simulink model "simulink"  (R2022b)
settings: Solver=VariableStepAuto  StartTime=0.0  StopTime=20  RelTol=1e-3
settings Model: Creator=25035  LastModifiedBy=ROG
settings ModelReferenceCC: EnableRefExpFcnMdlSchedulingChecks=on

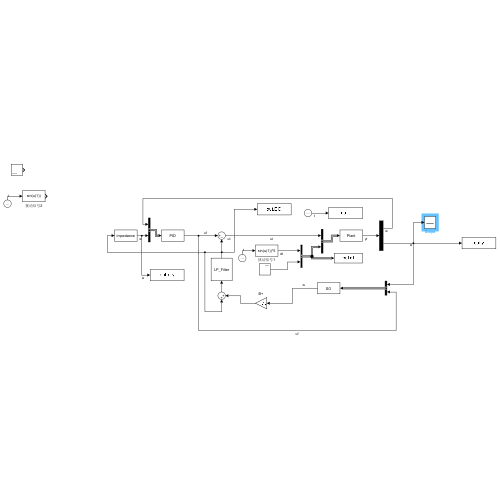
[thumbnail: Simulink's stored preview of the top-level diagram]
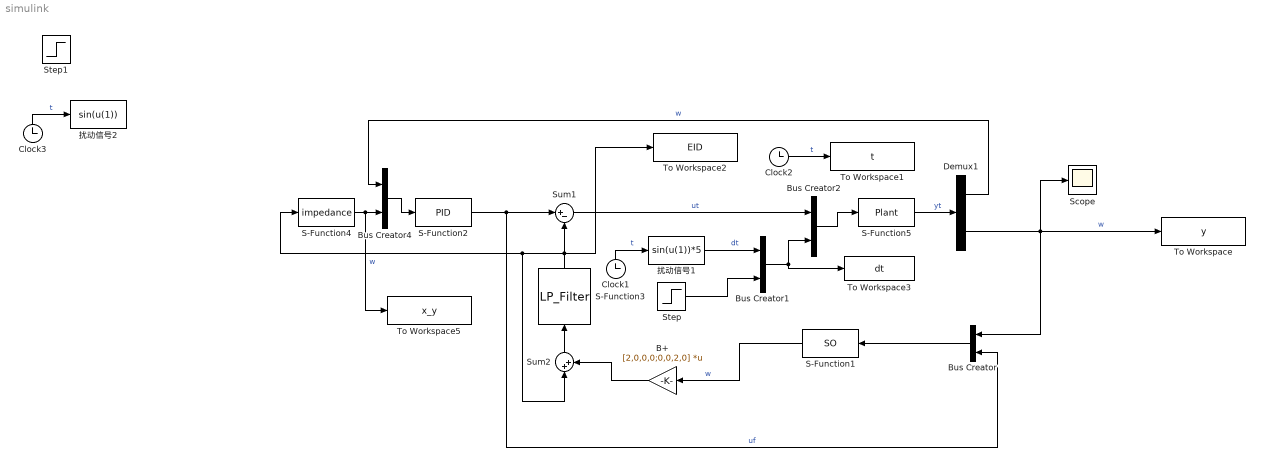
== system simulink ==
  B+ : Gain  Gain=[2,0,0,0;0,0,2,0]  Multiplication=Matrix(K*u)
  Bus Creator{,1..2,4} (4 alike) : BusCreator  Inputs=2
  Clock1 : Clock
  Clock2 : Clock
      settings: Decimation=30
  Clock3 : Clock
  Demux1 : Demux  Outputs=2
  S-Function1 : S-Function  FunctionName=SO  Parameters=PM  SFunctionDeploymentMode=off  EnableBusSupport=off
  S-Function2 : S-Function  FunctionName=PID  Parameters=PM  SFunctionDeploymentMode=off  EnableBusSupport=off
  S-Function3 : S-Function  FunctionName=LP_Filter  Parameters=PM  SFunctionDeploymentMode=off  EnableBusSupport=off
  S-Function4 : S-Function  FunctionName=impedance  Parameters=PM  SFunctionDeploymentMode=off  EnableBusSupport=off
  S-Function5 : S-Function  FunctionName=Plant  Parameters=PM  SFunctionDeploymentMode=off  EnableBusSupport=off
  Scope : Scope
  Step : Step  Time=0  SampleTime=0
  Step1 : Step  Time=0  SampleTime=0
  Sum1 : Sum  Inputs=|+-
  Sum2 : Sum  Inputs=|++
  To Workspace : ToWorkspace  VariableName=y  SampleTime=-1
  To Workspace1 : ToWorkspace  VariableName=t  SampleTime=-1
  To Workspace2 : ToWorkspace  VariableName=EID  SampleTime=-1
  To Workspace3 : ToWorkspace  VariableName=dt  SampleTime=-1
  To Workspace5 : ToWorkspace  VariableName=x_y  SampleTime=-1
  扰动信号1 : Fcn  Expr=sin(u(1))*5
  扰动信号2 : Fcn  Expr=sin(u(1))
  wires:
  S-Function2/1 -> Bus Creator/2, Sum1/1  "uf"
  S-Function3/1 -> To Workspace2/1, Sum1/2, Sum2/1, S-Function4/1
  Sum1/1 -> Bus Creator2/1  "ut"
  Bus Creator/1 -> S-Function1/1
  Sum2/1 -> S-Function3/1
  Bus Creator2/1 -> S-Function5/1
  Clock2/1 -> To Workspace1/1  "t"
  B+/1 -> Sum2/2
  S-Function1/1 -> B+/1  "w"
  Clock3/1 -> 扰动信号2/1  "t"
  S-Function5/1 -> Demux1/1  "yt"
  Demux1/1 -> Bus Creator4/1  "w"
  Clock1/1 -> 扰动信号1/1  "t"
  Bus Creator1/1 -> Bus Creator2/2, To Workspace3/1
  Bus Creator4/1 -> S-Function2/1
  Demux1/2 -> To Workspace/1, Bus Creator/1, Scope/1  "w"
  S-Function4/1 -> To Workspace5/1, Bus Creator4/2  "w"
  扰动信号1/1 -> Bus Creator1/1  "dt"
  Step/1 -> Bus Creator1/2
